simulink model "observe"  (R2021b)
settings: Solver=VariableStepAuto  StartTime=0.0  StopTime=20  RelTol=1e-3
settings Model: Creator=84232  LastModifiedBy=84232

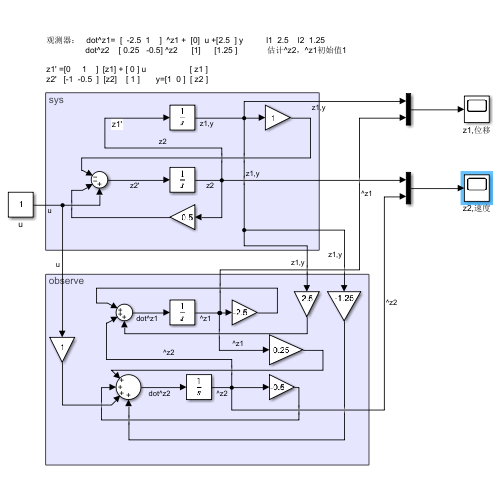
[thumbnail: Simulink's stored preview of the top-level diagram]
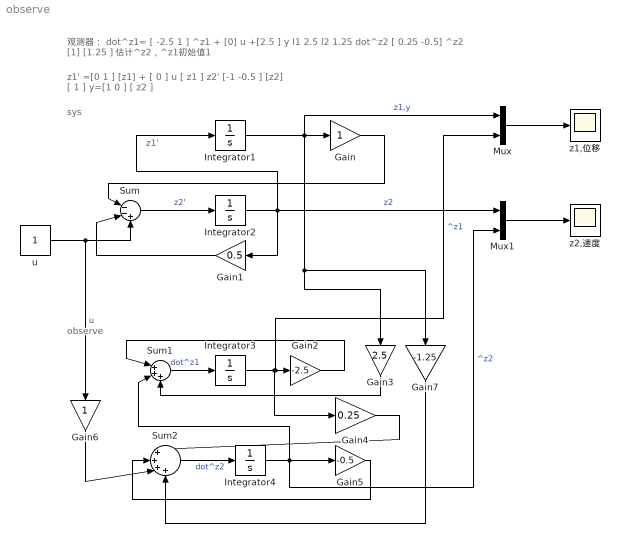
== system observe ==
  note: 观测器：   dot^z1=  [  -2.5  1    ]  ^z1 +  [0]  u +[2.5  ] y          l1  2.5    l2  1.25
      |                  dot^z2    [ 0.25   -0.5] ^z2      [1]      [1.25 ]             估计^z2，^z1初始值1
  note: observe
  note: z1' =[0     1    ]  [z1] + [ 0 ] u                   [ z1 ]
      | z2'   [-1  -0.5  ]  [z2]    [ 1 ]       y=[1  0 ]  [ z2 ]
  note: sys
  note: z1'
  Gain : Gain
  Gain1 : Gain  Gain=0.5
  Gain2 : Gain  Gain=-2.5
  Gain3 : Gain  Gain=2.5
  Gain4 : Gain  Gain=0.25
  Gain5 : Gain  Gain=-0.5
  Gain6 : Gain
  Gain7 : Gain  Gain=-1.25
  Integrator1 : Integrator
  Integrator2 : Integrator
  Integrator3 : Integrator  InitialCondition=1
  Integrator4 : Integrator  InitialCondition=1
  Mux : Mux  Inputs=2
  Mux1 : Mux  Inputs=2
  Sum : Sum  Inputs=|--+
  Sum1 : Sum  Inputs=|+++
  Sum2 : Sum  Inputs=|++++
  u : Constant
  z1,位移 : Scope
  z2,速度 : Scope
  wires:
  Integrator2/1 -> Integrator1/1, Mux1/1, Gain1/1  "z2"
  Sum/1 -> Integrator2/1  "z2'"
  Integrator1/1 -> Mux/1, Gain7/1, Gain3/1, Gain/1  "z1,y"
  Gain/1 -> Sum/1
  Gain1/1 -> Sum/2
  u/1 -> Gain6/1, Sum/3  "u"
  Integrator3/1 -> Gain4/1, Mux/2, Gain2/1  "^z1"
  Sum1/1 -> Integrator3/1  "dot^z1"
  Integrator4/1 -> Mux1/2, Gain5/1, Sum1/2  "^z2"
  Sum2/1 -> Integrator4/1  "dot^z2"
  Gain2/1 -> Sum1/1
  Gain3/1 -> Sum1/3
  Gain4/1 -> Sum2/1
  Gain5/1 -> Sum2/2
  Gain6/1 -> Sum2/3
  Gain7/1 -> Sum2/4
  Mux/1 -> z1,位移/1
  Mux1/1 -> z2,速度/1
